simulink model "Consolidate_state_feedback"  (Simulink 8.6)
settings: Solver=ode45  StartTime=0.0  StopTime=5  MaxStep=.00001  RelTol=1e-3
values from neighbouring files (symbols this model uses):
  A = [0 1; -50 -15]    [consolidated_models.m]
  B = [0;1]    [consolidated_models.m]
  C = [1 0]    [consolidated_models.m]
  K = acker(A, B, [-20 -25])    [consolidated_models.m]
settings Model: Creator=DR_C  LastModifiedBy=DR_C
settings DebuggingCC: FcnCallInpInsideContextMsg=EnableAllAsWarning
settings GRTTargetCC: CombineOutputUpdateFcns=on  GRTInterface=off

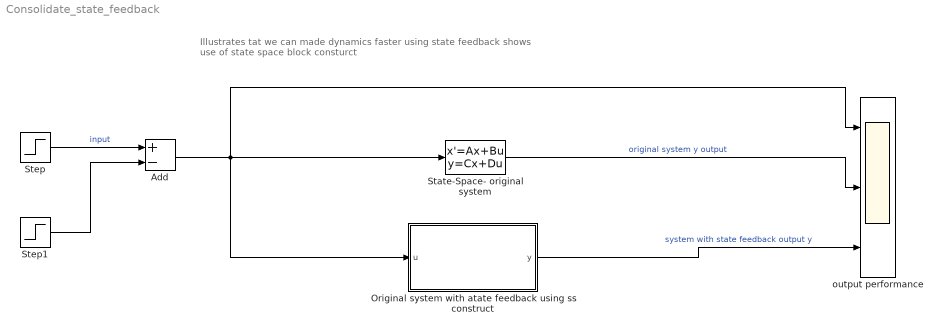
== system Consolidate_state_feedback ==
  note: Illustrates tat  we can made dynamics faster using state feedback
      | shows use of state space block consturct
  Add : Sum  Inputs=+-
  Original system with atate feedback using ss construct : Subsystem
  State-Space- original system : StateSpace  A=A  B=B  C=C  D=0  X0=0
  Step : Step  SampleTime=0
  Step1 : Step  Time=2  SampleTime=0
  output performance : Scope  NumInputPorts=3
  wires:
  State-Space- original system/1 -> output performance/2  "original system y output"
  Original system with atate feedback using ss construct/1(y) -> output performance/3  "system with state feedback output y"
  Step/1 -> Add/1  "input"
  Step1/1 -> Add/2
  Add/1 -> Original system with atate feedback using ss construct/1(u), output performance/1, State-Space- original system/1

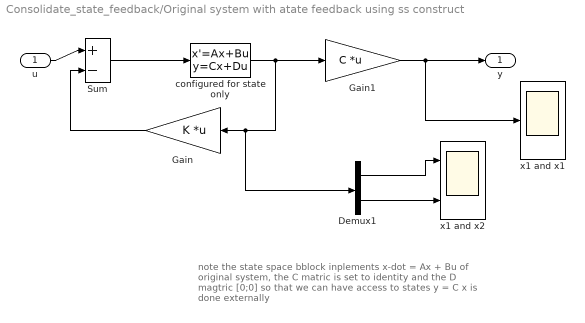
== system Consolidate_state_feedback/Original system with atate feedback using ss construct ==
  note: note the state space bblock
      | inplements x-dot = Ax + Bu of original
      | system, the C matric is set to identity and
      | the D magtric [0;0] so that we can have access to states
      | y = C x is done externally
  u : Inport
  Demux1 : Demux  Outputs=2
  Gain : Gain  Gain=K  Multiplication=Matrix(K*u) (u vector)
  Gain1 : Gain  Gain=C  Multiplication=Matrix(K*u) (u vector)
  Sum : Sum  Inputs=|+-
  configured for state only : StateSpace  A=A  B=B  C=eye(2)  D=[0;0]  X0=0
  x1 and x1 : Scope
  x1 and x2 : Scope  NumInputPorts=2
  y : Outport
  wires:
  Sum/1 -> configured for state only/1
  Gain/1 -> Sum/2
  configured for state only/1 -> Gain1/1, Gain/1, Demux1/1
  u/1 -> Sum/1
  Gain1/1 -> y/1, x1 and x1/1
  Demux1/1 -> x1 and x2/1
  Demux1/2 -> x1 and x2/2
